simulink model "robotarm"  (Simulink 6.3)
settings: Solver=ode45  StartTime=0.0  StopTime=10.0  RelTol=1e-3
settings Model: Creator=mbharadw  LastModifiedBy=mbharadw  ExtModeTrigMode=oneshot  ExtModeArmWhenConnect=off  StrictBusMsg=None
settings DataIOCC: LimitDataPoints=off
settings OptimizationCC: BlockReduction=off  BooleanDataType=off
settings DebuggingCC: SolverPrmCheckMsg=none
settings HardwareCC: TargetUnknown=on

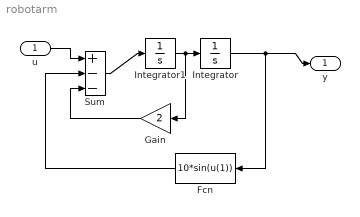
== system robotarm ==
  u : Inport
  Fcn : Fcn  Orientation=left  Expr=10*sin(u(1))
  Gain : Gain  Orientation=left  Gain=2  SaturateOnIntegerOverflow=on
  Integrator : Integrator
  Integrator1 : Integrator
  Sum : Sum  Inputs=+--  SaturateOnIntegerOverflow=on  InputSameDT=on
  y : Outport
  wires:
  Integrator/1 -> y/1, Fcn/1
  u/1 -> Sum/1
  Sum/1 -> Integrator1/1
  Fcn/1 -> Sum/2
  Integrator1/1 -> Integrator/1, Gain/1
  Gain/1 -> Sum/3
